simulink model "inverted_pendulum_model"  (R2020b)
settings: Solver=VariableStepAuto  StartTime=0.0  StopTime=10.0  RelTol=1e-3
settings Model: Creator=Mr Li  LastModifiedBy=Mr Li

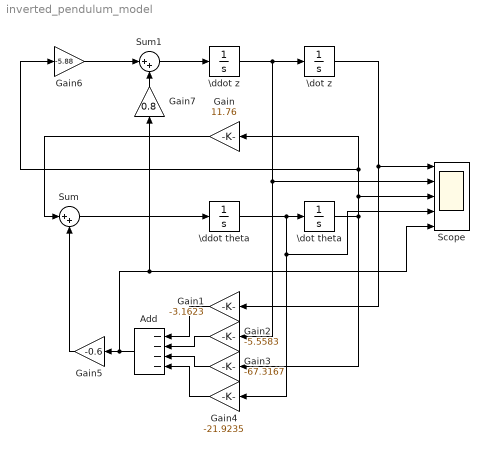
== system inverted_pendulum_model ==
  Add : Sum  Inputs=----
  Gain : Gain  Gain=11.76
  Gain1 : Gain  Gain=-3.1623
  Gain2 : Gain  Gain=-5.5583
  Gain3 : Gain  Gain=-67.3167
  Gain4 : Gain  Gain=-21.9235
  Gain5 : Gain  Gain=-0.6
  Gain6 : Gain  Gain=-5.88
  Gain7 : Gain  Gain=0.8
  Scope : Scope  NumInputPorts=5
  Sum : Sum  Inputs=|++
  Sum1 : Sum  Inputs=|++
  \ddot theta : Integrator
  \ddot z : Integrator
  \dot theta : Integrator  InitialCondition=0.5
  \dot z : Integrator
  wires:
  \ddot z/1 -> Gain2/1, Scope/2, \dot z/1
  \ddot theta/1 -> Scope/4, Gain4/1, \dot theta/1
  Sum/1 -> \ddot theta/1
  \dot theta/1 -> Gain6/1, Gain/1, Scope/3, Gain3/1
  Gain/1 -> Sum/1
  Gain2/1 -> Add/2
  Gain3/1 -> Add/3
  Gain1/1 -> Add/1
  Gain4/1 -> Add/4
  \dot z/1 -> Gain1/1, Scope/1
  Add/1 -> Scope/5, Gain7/1, Gain5/1
  Gain5/1 -> Sum/2
  Gain6/1 -> Sum1/1
  Sum1/1 -> \ddot z/1
  Gain7/1 -> Sum1/2
